simulink model "single_example"  (R2020a)
settings: Solver=VariableStepAuto  StartTime=0.0  StopTime=60  RelTol=1e-3
settings Model: Creator=aeagr  LastModifiedBy=aeagr

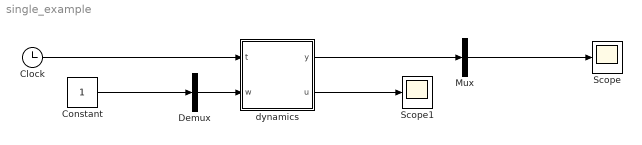
== system single_example ==
  Clock : Clock
  Constant : Constant
  Demux : Demux  Outputs=1
  Mux : Mux  Inputs=1
  Scope : Scope
  Scope1 : Scope
  dynamics : Subsystem
  wires:
  Clock/1 -> dynamics/1(t)
  Constant/1 -> Demux/1
  dynamics/1(y) -> Mux/1
  Demux/1 -> dynamics/2(w)
  Mux/1 -> Scope/1
  dynamics/2(u) -> Scope1/1

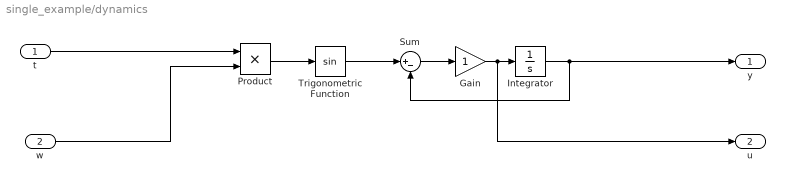
== system single_example/dynamics ==
  t : Inport
  w : Inport  Port=2
  Gain : Gain
  Integrator : Integrator
  Product : Product
  Sum : Sum  Inputs=|+-
  Trigonometric Function : Trigonometry
  y : Outport
  u : Outport  Port=2
  wires:
  Integrator/1 -> y/1, Sum/2
  w/1 -> Product/2
  Gain/1 -> u/1, Integrator/1
  Sum/1 -> Gain/1
  Product/1 -> Trigonometric Function/1
  Trigonometric Function/1 -> Sum/1
  t/1 -> Product/1
